simulink model "CSE_STEPRESPONSE_BLOCKDIAGRAM_NO6_DIPASUPIL"  (R2023a)
settings: Solver=VariableStepAuto  StartTime=0.0  StopTime=20.0  RelTol=1e-3
values from neighbouring files (symbols this model uses):
  G_den6 = [t u v w x]    [CSE_STEPRESPONSE_CODE_NO5_NO6_DIPASUPIL.m]    (also in CSE_STEPRESPONSE_CODE_NO6_DIPASUPIL.m)
  G_num6 = [p q r s]    [CSE_STEPRESPONSE_CODE_NO5_NO6_DIPASUPIL.m]    (also in CSE_STEPRESPONSE_CODE_NO6_DIPASUPIL.m)
settings Model: Creator=USER  LastModifiedBy=USER

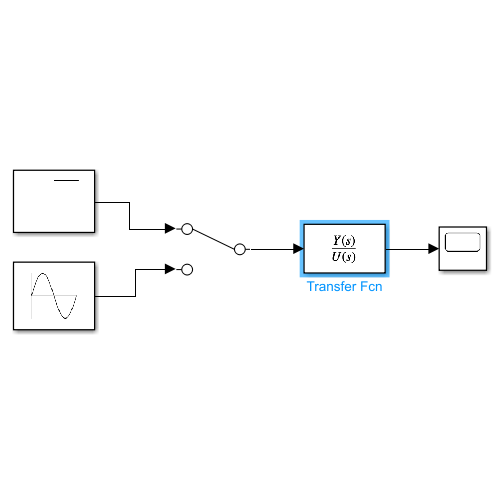
[thumbnail: Simulink's stored preview of the top-level diagram]
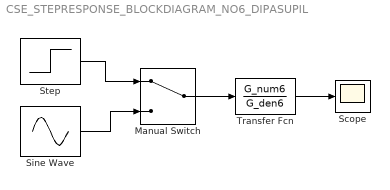
== system CSE_STEPRESPONSE_BLOCKDIAGRAM_NO6_DIPASUPIL ==
  Manual Switch : ManualSwitch
  Scope : Scope
  Sine Wave : Sin  SampleTime=0
  Step : Step  Time=0  SampleTime=0
  Transfer Fcn : TransferFcn  Numerator=G_num6  Denominator=G_den6
  wires:
  Step/1 -> Manual Switch/1
  Sine Wave/1 -> Manual Switch/2
  Manual Switch/1 -> Transfer Fcn/1
  Transfer Fcn/1 -> Scope/1
